simulink model "Enabled1"  (R2020a)
settings: Solver=VariableStepAuto  StartTime=0.0  StopTime=20  RelTol=1e-3
settings Model: Creator=BEAR  LastModifiedBy=bzhan
settings DataIOCC: ReturnWorkspaceOutputs=off
settings DebuggingCC: ArithmeticOperatorsInVariantConditions=warning
settings SFSimCC: SimUseLocalCustomCode=off  CustomCodeUndefinedFunction=UseInterfaceOnly
settings RTWCC: RTWUseLocalCustomCode=off

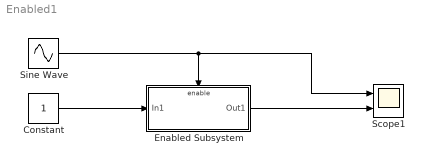
== system Enabled1 ==
  Constant : Constant
  Enabled Subsystem : Subsystem  TreatAsAtomicUnit=on
  Scope1 : Scope  NumInputPorts=2
  Sine Wave : Sin  SampleTime=0
  wires:
  Sine Wave/1 -> Scope1/1, Enabled Subsystem/Enable
  Constant/1 -> Enabled Subsystem/1(In1)
  Enabled Subsystem/1(Out1) -> Scope1/2

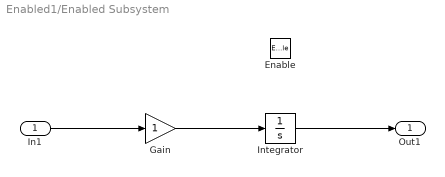
== system Enabled1/Enabled Subsystem ==
  In1 : Inport
  Enable : EnablePort
  Gain : Gain  SampleTime=2
  Integrator : Integrator
  Out1 : Outport  VectorParamsAs1DForOutWhenUnconnected=off
  wires:
  Integrator/1 -> Out1/1
  In1/1 -> Gain/1
  Gain/1 -> Integrator/1
